simulink model "APPL_DriverFaultDetection"  (R2018b)
settings: configuration reference "CodeConfig_10_ms" (kept outside this file)
undefined symbols (not defined in the file): CAL_LockErrNoTime_30ms, CAL_ManualSwValid_90s, CAL_MotorHallInvalid_2s, CAL_MotorMaxRunTime_60s, CAL_MotorRelayErr_2s, CAL_MotorStall_750ms, D_DrSoftStopDef_B, D_DrSoftStopDef_F, D_DrSoftStopDef_H, D_DrSoftStopDef_L, D_Relay_DownBackFault, D_Relay_UpFrontFault, enSeatMoveCmd, FALSE, TRUE
libraries: DareLib x95, simulink x2
(part 2 of 3)

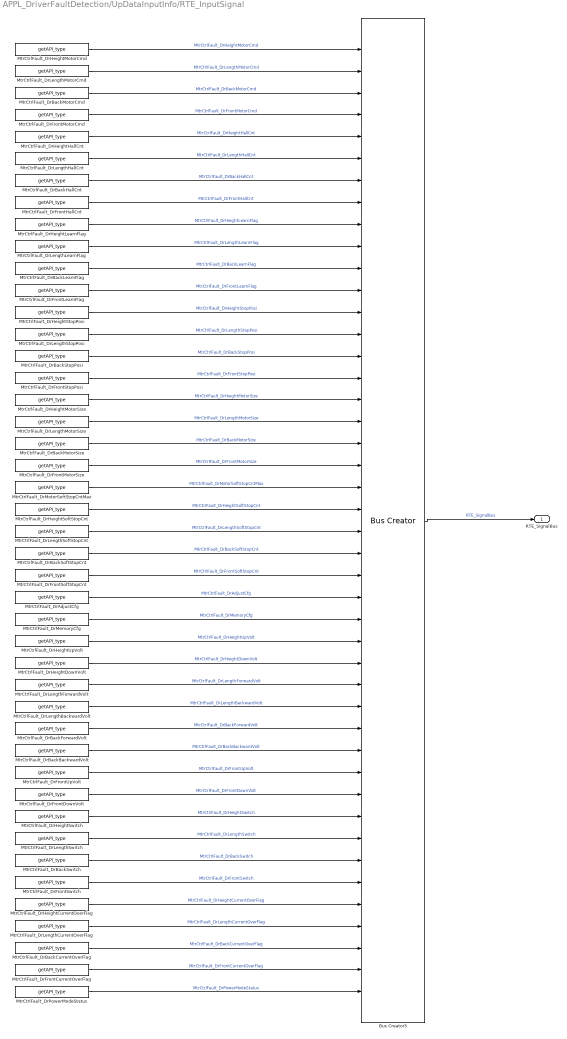
== system APPL_DriverFaultDetection/UpDataInputInfo/RTE_InputSignal ==
  Bus Creator5 : BusCreator  Inputs=44
  MtrCtrlFault_DrAdjustCfg : DareLib/Dare/getAPI_type  g_funcname=Srvl_GetMemIndexDataU8  g_param=EN_MemIndex_DrAdjustConfig  g_type=uint8  g_enum=enDrAdjustEnable  g_size=-1
      settings: AttributesFormatString=%<g_funcname>  SourceProductName=Dare Library
  MtrCtrlFault_DrBackBackwardVolt : DareLib/Dare/getAPI_type  g_funcname=Ecual_GetDrRelayFlagBackBackward  g_param=""  g_type=uint8  g_size=-1
      settings: AttributesFormatString=%<g_funcname>  SourceProductName=Dare Library
  MtrCtrlFault_DrBackCurrentOverFlag : DareLib/Dare/getAPI_type  g_funcname=Ecual_GetDrBackOverCurrentFlag  g_param=""  g_type=uint8  g_size=-1
      settings: AttributesFormatString=%<g_funcname>  SourceProductName=Dare Library
  MtrCtrlFault_DrBackForwardVolt : DareLib/Dare/getAPI_type  g_funcname=Ecual_GetDrRelayFlagBackForward  g_param=""  g_type=uint8  g_size=-1
      settings: AttributesFormatString=%<g_funcname>  SourceProductName=Dare Library
  MtrCtrlFault_DrBackHallCnt : DareLib/Dare/getAPI_type  g_funcname=Cdd_GetCurrentHallCnt  g_param=EN_DriverBack  g_type=uint16  g_size=-1
      settings: AttributesFormatString=%<g_funcname>  SourceProductName=Dare Library
  MtrCtrlFault_DrBackLearnFlag : DareLib/Dare/getAPI_type  g_funcname=Cdd_GetMotorLearnFlag  g_param=EN_DriverBack  g_type=uint8  g_size=-1
      settings: AttributesFormatString=%<g_funcname>  SourceProductName=Dare Library
  MtrCtrlFault_DrBackMotorCmd : DareLib/Dare/getAPI_type  g_funcname=Rte_GetVfb_DrBackMotorCmd  g_param=""  g_type=uint8  g_size=-1
      settings: AttributesFormatString=%<g_funcname>  SourceProductName=Dare Library
  MtrCtrlFault_DrBackMotorSize : DareLib/Dare/getAPI_type  g_funcname=Cdd_GetMotorSize  g_param=EN_DriverBack  g_type=uint16  g_size=-1
      settings: AttributesFormatString=%<g_funcname>  SourceProductName=Dare Library
  MtrCtrlFault_DrBackSoftStopCnt : DareLib/Dare/getAPI_type  g_funcname=Srvl_GetMemIndexDataU8  g_param=EN_MemIndex_DrBackSoftStopCnt  g_type=uint8  g_size=-1
      settings: AttributesFormatString=%<g_funcname>  SourceProductName=Dare Library
  MtrCtrlFault_DrBackStopPosi : DareLib/Dare/getAPI_type  g_funcname=Cdd_GetMotorHardStop  g_param=EN_DriverBack  g_type=uint16  g_size=-1
      settings: AttributesFormatString=%<g_funcname>  SourceProductName=Dare Library
  MtrCtrlFault_DrBackSwitch : DareLib/Dare/getAPI_type  g_funcname=Ecual_GetDrBackSwitchCmd  g_param=""  g_type=uint8  g_enum=enSeatMoveCmd  g_size=-1
      settings: AttributesFormatString=%<g_funcname>  SourceProductName=Dare Library
  MtrCtrlFault_DrFrontCurrentOverFlag : DareLib/Dare/getAPI_type  g_funcname=Ecual_GetDrFrontOverCurrentFlag  g_param=""  g_type=uint8  g_size=-1
      settings: AttributesFormatString=%<g_funcname>  SourceProductName=Dare Library
  MtrCtrlFault_DrFrontDownVolt : DareLib/Dare/getAPI_type  g_funcname=Ecual_GetDrRelayFlagFrontDown  g_param=""  g_type=uint8  g_size=-1
      settings: AttributesFormatString=%<g_funcname>  SourceProductName=Dare Library
  MtrCtrlFault_DrFrontHallCnt : DareLib/Dare/getAPI_type  g_funcname=Cdd_GetCurrentHallCnt  g_param=EN_DriverFront  g_type=uint16  g_size=-1
      settings: AttributesFormatString=%<g_funcname>  SourceProductName=Dare Library
  MtrCtrlFault_DrFrontLearnFlag : DareLib/Dare/getAPI_type  g_funcname=Cdd_GetMotorLearnFlag  g_param=EN_DriverFront  g_type=uint8  g_size=-1
      settings: AttributesFormatString=%<g_funcname>  SourceProductName=Dare Library
  MtrCtrlFault_DrFrontMotorCmd : DareLib/Dare/getAPI_type  g_funcname=Rte_GetVfb_DrFrontMotorCmd  g_param=""  g_type=uint8  g_size=-1
      settings: AttributesFormatString=%<g_funcname>  SourceProductName=Dare Library
  MtrCtrlFault_DrFrontMotorSize : DareLib/Dare/getAPI_type  g_funcname=Cdd_GetMotorSize  g_param=EN_DriverFront  g_type=uint16  g_size=-1
      settings: AttributesFormatString=%<g_funcname>  SourceProductName=Dare Library
  MtrCtrlFault_DrFrontSoftStopCnt : DareLib/Dare/getAPI_type  g_funcname=Srvl_GetMemIndexDataU8  g_param=EN_MemIndex_DrFrontSoftStopCnt  g_type=uint8  g_size=-1
      settings: AttributesFormatString=%<g_funcname>  SourceProductName=Dare Library
  MtrCtrlFault_DrFrontStopPosi : DareLib/Dare/getAPI_type  g_funcname=Cdd_GetMotorHardStop  g_param=EN_DriverFront  g_type=uint16  g_size=-1
      settings: AttributesFormatString=%<g_funcname>  SourceProductName=Dare Library
  MtrCtrlFault_DrFrontSwitch : DareLib/Dare/getAPI_type  g_funcname=Ecual_GetDrFrontSwitchCmd  g_param=""  g_type=uint8  g_enum=enSeatMoveCmd  g_size=-1
      settings: AttributesFormatString=%<g_funcname>  SourceProductName=Dare Library
  MtrCtrlFault_DrFrontUpVolt : DareLib/Dare/getAPI_type  g_funcname=Ecual_GetDrRelayFlagFrontUp  g_param=""  g_type=uint8  g_size=-1
      settings: AttributesFormatString=%<g_funcname>  SourceProductName=Dare Library
  MtrCtrlFault_DrHeightCurrentOverFlag : DareLib/Dare/getAPI_type  g_funcname=Ecual_GetDrHeightOverCurrentFlag  g_param=""  g_type=uint8  g_size=-1
      settings: AttributesFormatString=%<g_funcname>  SourceProductName=Dare Library
  MtrCtrlFault_DrHeightDownVolt : DareLib/Dare/getAPI_type  g_funcname=Ecual_GetDrRelayFlagHeightDN  g_param=""  g_type=uint8  g_size=-1
      settings: AttributesFormatString=%<g_funcname>  SourceProductName=Dare Library
  MtrCtrlFault_DrHeightHallCnt : DareLib/Dare/getAPI_type  g_funcname=Cdd_GetCurrentHallCnt  g_param=EN_DriverHeight  g_type=uint16  g_size=-1
      settings: AttributesFormatString=%<g_funcname>  SourceProductName=Dare Library
  MtrCtrlFault_DrHeightLearnFlag : DareLib/Dare/getAPI_type  g_funcname=Cdd_GetMotorLearnFlag  g_param=EN_DriverHeight  g_type=uint8  g_size=-1
      settings: AttributesFormatString=%<g_funcname>  SourceProductName=Dare Library
  MtrCtrlFault_DrHeightMotorCmd : DareLib/Dare/getAPI_type  g_funcname=Rte_GetVfb_DrHeightMotorCmd  g_param=""  g_type=uint8  g_size=-1
      settings: AttributesFormatString=%<g_funcname>  SourceProductName=Dare Library
  MtrCtrlFault_DrHeightMotorSize : DareLib/Dare/getAPI_type  g_funcname=Cdd_GetMotorSize  g_param=EN_DriverHeight  g_type=uint16  g_size=-1
      settings: AttributesFormatString=%<g_funcname>  SourceProductName=Dare Library
  MtrCtrlFault_DrHeightSoftStopCnt : DareLib/Dare/getAPI_type  g_funcname=Srvl_GetMemIndexDataU8  g_param=EN_MemIndex_DrHeightSoftStopCnt  g_type=uint8  g_size=-1
      settings: AttributesFormatString=%<g_funcname>  SourceProductName=Dare Library
  MtrCtrlFault_DrHeightStopPosi : DareLib/Dare/getAPI_type  g_funcname=Cdd_GetMotorHardStop  g_param=EN_DriverHeight  g_type=uint16  g_size=-1
      settings: AttributesFormatString=%<g_funcname>  SourceProductName=Dare Library
  MtrCtrlFault_DrHeightSwitch : DareLib/Dare/getAPI_type  g_funcname=Ecual_GetDrHeightSwitchCmd  g_param=""  g_type=uint8  g_enum=enSeatMoveCmd  g_size=-1
      settings: AttributesFormatString=%<g_funcname>  SourceProductName=Dare Library
  MtrCtrlFault_DrHeightUpVolt : DareLib/Dare/getAPI_type  g_funcname=Ecual_GetDrRelayFlagHeightUp  g_param=""  g_type=uint8  g_size=-1
      settings: AttributesFormatString=%<g_funcname>  SourceProductName=Dare Library
  MtrCtrlFault_DrLengthBackwardVolt : DareLib/Dare/getAPI_type  g_funcname=Ecual_GetDrRelayFlagLenghtBackward  g_param=""  g_type=uint8  g_size=-1
      settings: AttributesFormatString=%<g_funcname>  SourceProductName=Dare Library
  MtrCtrlFault_DrLengthCurrentOverFlag : DareLib/Dare/getAPI_type  g_funcname=Ecual_GetDrLengthOverCurrentFlag  g_param=""  g_type=uint8  g_size=-1
      settings: AttributesFormatString=%<g_funcname>  SourceProductName=Dare Library
  MtrCtrlFault_DrLengthForwardVolt : DareLib/Dare/getAPI_type  g_funcname=Ecual_GetDrRelayFlagLenghtForward  g_param=""  g_type=uint8  g_size=-1
      settings: AttributesFormatString=%<g_funcname>  SourceProductName=Dare Library
  MtrCtrlFault_DrLengthHallCnt : DareLib/Dare/getAPI_type  g_funcname=Cdd_GetCurrentHallCnt  g_param=EN_DriverLength  g_type=uint16  g_size=-1
      settings: AttributesFormatString=%<g_funcname>  SourceProductName=Dare Library
  MtrCtrlFault_DrLengthLearnFlag : DareLib/Dare/getAPI_type  g_funcname=Cdd_GetMotorLearnFlag  g_param=EN_DriverLength  g_type=uint8  g_size=-1
      settings: AttributesFormatString=%<g_funcname>  SourceProductName=Dare Library
  MtrCtrlFault_DrLengthMotorCmd : DareLib/Dare/getAPI_type  g_funcname=Rte_GetVfb_DrLengthMotorCmd  g_param=""  g_type=uint8  g_size=-1
      settings: AttributesFormatString=%<g_funcname>  SourceProductName=Dare Library
  MtrCtrlFault_DrLengthMotorSize : DareLib/Dare/getAPI_type  g_funcname=Cdd_GetMotorSize  g_param=EN_DriverLength  g_type=uint16  g_size=-1
      settings: AttributesFormatString=%<g_funcname>  SourceProductName=Dare Library
  MtrCtrlFault_DrLengthSoftStopCnt : DareLib/Dare/getAPI_type  g_funcname=Srvl_GetMemIndexDataU8  g_param=EN_MemIndex_DrLengthSoftStopCnt  g_type=uint8  g_size=-1
      settings: AttributesFormatString=%<g_funcname>  SourceProductName=Dare Library
  MtrCtrlFault_DrLengthStopPosi : DareLib/Dare/getAPI_type  g_funcname=Cdd_GetMotorHardStop  g_param=EN_DriverLength  g_type=uint16  g_size=-1
      settings: AttributesFormatString=%<g_funcname>  SourceProductName=Dare Library
  MtrCtrlFault_DrLengthSwitch : DareLib/Dare/getAPI_type  g_funcname=Ecual_GetDrLengthSwitchCmd  g_param=""  g_type=uint8  g_enum=enSeatMoveCmd  g_size=-1
      settings: AttributesFormatString=%<g_funcname>  SourceProductName=Dare Library
  MtrCtrlFault_DrMemoryCfg : DareLib/Dare/getAPI_type  g_funcname=Srvl_GetMemIndexDataU8  g_param=EN_MemIndex_DrMemoryConfig  g_type=uint8  g_size=-1
      settings: AttributesFormatString=%<g_funcname>  SourceProductName=Dare Library
  MtrCtrlFault_DrMotorSoftStopCntMax : DareLib/Dare/getAPI_type  g_funcname=Srvl_GetMemIndexDataU8  g_param=EN_MemIndex_MotorSoftStopCntMax  g_type=uint8  g_size=-1
      settings: AttributesFormatString=%<g_funcname>  SourceProductName=Dare Library
  MtrCtrlFault_DrPowerModeStatus : DareLib/Dare/getAPI_type  g_funcname=Rte_GetVfb_PowerMode  g_param=""  g_type=uint8  g_enum=enIgnSts  g_size=-1
      settings: AttributesFormatString=%<g_funcname>  SourceProductName=Dare Library
  RTE_SignalBus : Outport
  wires:
  Bus Creator5/1 -> RTE_SignalBus/1  "RTE_SignalBus"
  MtrCtrlFault_DrHeightMotorCmd/1 -> Bus Creator5/1  "MtrCtrlFault_DrHeightMotorCmd"
  MtrCtrlFault_DrLengthMotorCmd/1 -> Bus Creator5/2  "MtrCtrlFault_DrLengthMotorCmd"
  MtrCtrlFault_DrBackMotorCmd/1 -> Bus Creator5/3  "MtrCtrlFault_DrBackMotorCmd"
  MtrCtrlFault_DrFrontMotorCmd/1 -> Bus Creator5/4  "MtrCtrlFault_DrFrontMotorCmd"
  MtrCtrlFault_DrHeightHallCnt/1 -> Bus Creator5/5  "MtrCtrlFault_DrHeightHallCnt"
  MtrCtrlFault_DrLengthHallCnt/1 -> Bus Creator5/6  "MtrCtrlFault_DrLengthHallCnt"
  MtrCtrlFault_DrBackHallCnt/1 -> Bus Creator5/7  "MtrCtrlFault_DrBackHallCnt"
  MtrCtrlFault_DrFrontHallCnt/1 -> Bus Creator5/8  "MtrCtrlFault_DrFrontHallCnt"
  MtrCtrlFault_DrHeightLearnFlag/1 -> Bus Creator5/9  "MtrCtrlFault_DrHeightLearnFlag"
  MtrCtrlFault_DrLengthLearnFlag/1 -> Bus Creator5/10  "MtrCtrlFault_DrLengthLearnFlag"
  MtrCtrlFault_DrBackLearnFlag/1 -> Bus Creator5/11  "MtrCtrlFault_DrBackLearnFlag"
  MtrCtrlFault_DrFrontLearnFlag/1 -> Bus Creator5/12  "MtrCtrlFault_DrFrontLearnFlag"
  MtrCtrlFault_DrHeightStopPosi/1 -> Bus Creator5/13  "MtrCtrlFault_DrHeightStopPosi"
  MtrCtrlFault_DrLengthStopPosi/1 -> Bus Creator5/14  "MtrCtrlFault_DrLengthStopPosi"
  MtrCtrlFault_DrBackStopPosi/1 -> Bus Creator5/15  "MtrCtrlFault_DrBackStopPosi"
  MtrCtrlFault_DrFrontStopPosi/1 -> Bus Creator5/16  "MtrCtrlFault_DrFrontStopPosi"
  MtrCtrlFault_DrHeightMotorSize/1 -> Bus Creator5/17  "MtrCtrlFault_DrHeightMotorSize"
  MtrCtrlFault_DrLengthMotorSize/1 -> Bus Creator5/18  "MtrCtrlFault_DrLengthMotorSize"
  MtrCtrlFault_DrBackMotorSize/1 -> Bus Creator5/19  "MtrCtrlFault_DrBackMotorSize"
  MtrCtrlFault_DrFrontMotorSize/1 -> Bus Creator5/20  "MtrCtrlFault_DrFrontMotorSize"
  MtrCtrlFault_DrMotorSoftStopCntMax/1 -> Bus Creator5/21  "MtrCtrlFault_DrMotorSoftStopCntMax"
  MtrCtrlFault_DrHeightSoftStopCnt/1 -> Bus Creator5/22  "MtrCtrlFault_DrHeightSoftStopCnt"
  MtrCtrlFault_DrLengthSoftStopCnt/1 -> Bus Creator5/23  "MtrCtrlFault_DrLengthSoftStopCnt"
  MtrCtrlFault_DrBackSoftStopCnt/1 -> Bus Creator5/24  "MtrCtrlFault_DrBackSoftStopCnt"
  MtrCtrlFault_DrFrontSoftStopCnt/1 -> Bus Creator5/25  "MtrCtrlFault_DrFrontSoftStopCnt"
  MtrCtrlFault_DrAdjustCfg/1 -> Bus Creator5/26  "MtrCtrlFault_DrAdjustCfg"
  MtrCtrlFault_DrMemoryCfg/1 -> Bus Creator5/27  "MtrCtrlFault_DrMemoryCfg"
  MtrCtrlFault_DrHeightUpVolt/1 -> Bus Creator5/28  "MtrCtrlFault_DrHeightUpVolt"
  MtrCtrlFault_DrHeightDownVolt/1 -> Bus Creator5/29  "MtrCtrlFault_DrHeightDownVolt"
  MtrCtrlFault_DrLengthForwardVolt/1 -> Bus Creator5/30  "MtrCtrlFault_DrLengthForwardVolt"
  MtrCtrlFault_DrLengthBackwardVolt/1 -> Bus Creator5/31  "MtrCtrlFault_DrLengthBackwardVolt"
  MtrCtrlFault_DrBackForwardVolt/1 -> Bus Creator5/32  "MtrCtrlFault_DrBackForwardVolt"
  MtrCtrlFault_DrBackBackwardVolt/1 -> Bus Creator5/33  "MtrCtrlFault_DrBackBackwardVolt"
  MtrCtrlFault_DrFrontUpVolt/1 -> Bus Creator5/34  "MtrCtrlFault_DrFrontUpVolt"
  MtrCtrlFault_DrFrontDownVolt/1 -> Bus Creator5/35  "MtrCtrlFault_DrFrontDownVolt"
  MtrCtrlFault_DrHeightSwitch/1 -> Bus Creator5/36  "MtrCtrlFault_DrHeightSwitch"
  MtrCtrlFault_DrLengthSwitch/1 -> Bus Creator5/37  "MtrCtrlFault_DrLengthSwitch"
  MtrCtrlFault_DrBackSwitch/1 -> Bus Creator5/38  "MtrCtrlFault_DrBackSwitch"
  MtrCtrlFault_DrFrontSwitch/1 -> Bus Creator5/39  "MtrCtrlFault_DrFrontSwitch"
  MtrCtrlFault_DrHeightCurrentOverFlag/1 -> Bus Creator5/40  "MtrCtrlFault_DrHeightCurrentOverFlag"
  MtrCtrlFault_DrLengthCurrentOverFlag/1 -> Bus Creator5/41  "MtrCtrlFault_DrLengthCurrentOverFlag"
  MtrCtrlFault_DrBackCurrentOverFlag/1 -> Bus Creator5/42  "MtrCtrlFault_DrBackCurrentOverFlag"
  MtrCtrlFault_DrFrontCurrentOverFlag/1 -> Bus Creator5/43  "MtrCtrlFault_DrFrontCurrentOverFlag"
  MtrCtrlFault_DrPowerModeStatus/1 -> Bus Creator5/44  "MtrCtrlFault_DrPowerModeStatus"

== system APPL_DriverFaultDetection/LogicCtrl/AdheAndEffec/SwitchErrorDetection/GetCurMsTs ==
  f : TriggerPort  TriggerType=function-call  VariantControl=(inherit)
      settings: CopyFcn=Stateflow.SLINSF.SimulinkMan.removeBlockPreDeleteFcn  PreDeleteFcn=Stateflow.SLINSF.SimulinkMan.unsafePredeleteFcn
  DrAdj_LenAdjSize : DareLib/Dare/getAPI_type  g_funcname=D_HAL_GET_CUR_MS_TS  g_param=""  g_type=uint32  g_size=-1
      settings: SourceProductName=Dare Library
  Ts : Outport
  wires:
  DrAdj_LenAdjSize/1 -> Ts/1  "DrAdj_CurMsTs"

== system APPL_DriverFaultDetection/LogicCtrl/AdheAndEffec/SwitchErrorDetection/GetDefTime ==
  DefTs : Inport
  Ts : Inport  Port=2
  f : TriggerPort  TriggerType=function-call  VariantControl=(inherit)
      settings: CopyFcn=Stateflow.SLINSF.SimulinkMan.removeBlockPreDeleteFcn  PreDeleteFcn=Stateflow.SLINSF.SimulinkMan.unsafePredeleteFcn
  Chart : Stateflow chart  TreatAsAtomicUnit=on
  OutTs : Outport
  wires:
  DefTs/1 -> Chart/1(DefTs)
  Ts/1 -> Chart/2(Ts)
  Chart/1(OutTs) -> OutTs/1

== system APPL_DriverFaultDetection/LogicCtrl/AdheAndEffec/SwitchErrorDetection/TimeDiffTs ==
  lastTs : Inport
  Ts : Inport  Port=2
  f : TriggerPort  TriggerType=function-call  VariantControl=(inherit)
      settings: CopyFcn=Stateflow.SLINSF.SimulinkMan.removeBlockPreDeleteFcn  PreDeleteFcn=Stateflow.SLINSF.SimulinkMan.unsafePredeleteFcn
  Chart : Stateflow chart  TreatAsAtomicUnit=on
  OutTs : Outport
  wires:
  lastTs/1 -> Chart/1(lastTs)
  Ts/1 -> Chart/2(Ts)
  Chart/1(OutTs) -> OutTs/1

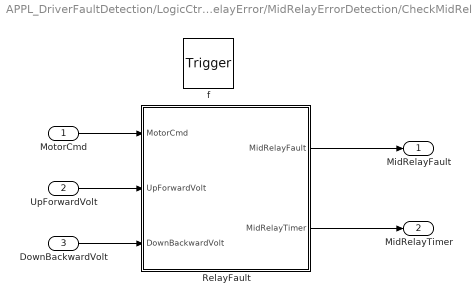
== system APPL_DriverFaultDetection/LogicCtrl/RelayError/MidRelayErrorDetection/CheckMidRelayFault ==
  MotorCmd : Inport  OutDataTypeStr=uint8  PortDimensions=1
  UpForwardVolt : Inport  Port=2  OutDataTypeStr=uint8  PortDimensions=1
  DownBackwardVolt : Inport  Port=3  OutDataTypeStr=uint8  PortDimensions=1
  f : TriggerPort  TriggerType=function-call  VariantControl=(inherit)
      settings: CopyFcn=Stateflow.SLINSF.SimulinkMan.removeBlockPreDeleteFcn  PreDeleteFcn=Stateflow.SLINSF.SimulinkMan.unsafePredeleteFcn
  RelayFault : Stateflow chart  TreatAsAtomicUnit=on
  MidRelayFault : Outport  OutDataTypeStr=uint8
  MidRelayTimer : Outport  Port=2  OutDataTypeStr=uint8
  wires:
  MotorCmd/1 -> RelayFault/1(MotorCmd)
  UpForwardVolt/1 -> RelayFault/2(UpForwardVolt)
  DownBackwardVolt/1 -> RelayFault/3(DownBackwardVolt)
  RelayFault/1(MidRelayFault) -> MidRelayFault/1
  RelayFault/2(MidRelayTimer) -> MidRelayTimer/1

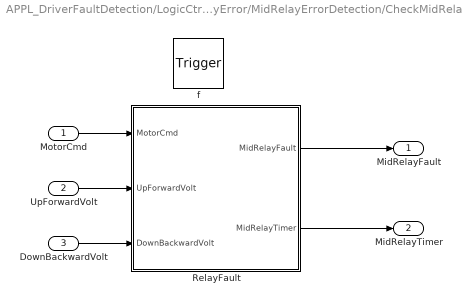
== system APPL_DriverFaultDetection/LogicCtrl/RelayError/MidRelayErrorDetection/CheckMidRelayFault1 ==
  MotorCmd : Inport  OutDataTypeStr=uint8  PortDimensions=1
  UpForwardVolt : Inport  Port=2  OutDataTypeStr=uint8  PortDimensions=1
  DownBackwardVolt : Inport  Port=3  OutDataTypeStr=uint8  PortDimensions=1
  f : TriggerPort  TriggerType=function-call  VariantControl=(inherit)
      settings: CopyFcn=Stateflow.SLINSF.SimulinkMan.removeBlockPreDeleteFcn  PreDeleteFcn=Stateflow.SLINSF.SimulinkMan.unsafePredeleteFcn
  RelayFault : Stateflow chart  TreatAsAtomicUnit=on
  MidRelayFault : Outport  OutDataTypeStr=uint8
  MidRelayTimer : Outport  Port=2  OutDataTypeStr=uint8
  wires:
  MotorCmd/1 -> RelayFault/1(MotorCmd)
  UpForwardVolt/1 -> RelayFault/2(UpForwardVolt)
  DownBackwardVolt/1 -> RelayFault/3(DownBackwardVolt)
  RelayFault/1(MidRelayFault) -> MidRelayFault/1
  RelayFault/2(MidRelayTimer) -> MidRelayTimer/1

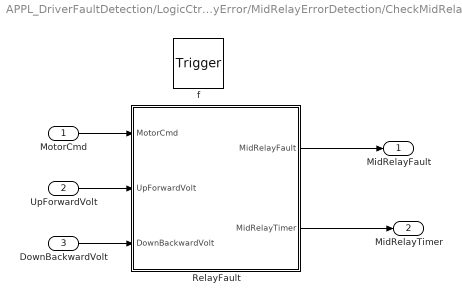
== system APPL_DriverFaultDetection/LogicCtrl/RelayError/MidRelayErrorDetection/CheckMidRelayFault2 ==
  MotorCmd : Inport  OutDataTypeStr=uint8  PortDimensions=1
  UpForwardVolt : Inport  Port=2  OutDataTypeStr=uint8  PortDimensions=1
  DownBackwardVolt : Inport  Port=3  OutDataTypeStr=uint8  PortDimensions=1
  f : TriggerPort  TriggerType=function-call  VariantControl=(inherit)
      settings: CopyFcn=Stateflow.SLINSF.SimulinkMan.removeBlockPreDeleteFcn  PreDeleteFcn=Stateflow.SLINSF.SimulinkMan.unsafePredeleteFcn
  RelayFault : Stateflow chart  TreatAsAtomicUnit=on
  MidRelayFault : Outport  OutDataTypeStr=uint8
  MidRelayTimer : Outport  Port=2  OutDataTypeStr=uint8
  wires:
  MotorCmd/1 -> RelayFault/1(MotorCmd)
  UpForwardVolt/1 -> RelayFault/2(UpForwardVolt)
  DownBackwardVolt/1 -> RelayFault/3(DownBackwardVolt)
  RelayFault/1(MidRelayFault) -> MidRelayFault/1
  RelayFault/2(MidRelayTimer) -> MidRelayTimer/1

== system APPL_DriverFaultDetection/LogicCtrl/RelayError/MidRelayErrorDetection/CheckMidRelayFault3 ==
  MotorCmd : Inport  OutDataTypeStr=uint8  PortDimensions=1
  UpForwardVolt : Inport  Port=2  OutDataTypeStr=uint8  PortDimensions=1
  DownBackwardVolt : Inport  Port=3  OutDataTypeStr=uint8  PortDimensions=1
  f : TriggerPort  TriggerType=function-call  VariantControl=(inherit)
      settings: CopyFcn=Stateflow.SLINSF.SimulinkMan.removeBlockPreDeleteFcn  PreDeleteFcn=Stateflow.SLINSF.SimulinkMan.unsafePredeleteFcn
  RelayFault : Stateflow chart  TreatAsAtomicUnit=on
  MidRelayFault : Outport  OutDataTypeStr=uint8
  MidRelayTimer : Outport  Port=2  OutDataTypeStr=uint8
  wires:
  MotorCmd/1 -> RelayFault/1(MotorCmd)
  UpForwardVolt/1 -> RelayFault/2(UpForwardVolt)
  DownBackwardVolt/1 -> RelayFault/3(DownBackwardVolt)
  RelayFault/1(MidRelayFault) -> MidRelayFault/1
  RelayFault/2(MidRelayTimer) -> MidRelayTimer/1

== system APPL_DriverFaultDetection/LogicCtrl/SoftStopPoint/SoftStopPointDetection/DrAdj_SetBackSoftStopCnt ==
  Cnt : Inport
  f : TriggerPort  TriggerType=function-call  VariantControl=(inherit)
      settings: CopyFcn=Stateflow.SLINSF.SimulinkMan.removeBlockPreDeleteFcn  PreDeleteFcn=Stateflow.SLINSF.SimulinkMan.unsafePredeleteFcn
  DriverFrontMoveType12 : DareLib/Dare/setAPI_type  g_funcname=Srvl_SetMemIndexDataU8  g_param=EN_MemIndex_DrBackSoftStopCnt  g_type=uint8  g_size=-1
      settings: AttributesFormatString=%<g_funcname>  SourceProductName=Dare Library
  wires:
  Cnt/1 -> DriverFrontMoveType12/1

== system APPL_DriverFaultDetection/LogicCtrl/SoftStopPoint/SoftStopPointDetection/DrAdj_SetFrontSoftStopCnt ==
  Cnt : Inport
  f : TriggerPort  TriggerType=function-call  VariantControl=(inherit)
      settings: CopyFcn=Stateflow.SLINSF.SimulinkMan.removeBlockPreDeleteFcn  PreDeleteFcn=Stateflow.SLINSF.SimulinkMan.unsafePredeleteFcn
  DriverFrontMoveType12 : DareLib/Dare/setAPI_type  g_funcname=Srvl_SetMemIndexDataU8  g_param=EN_MemIndex_DrFrontSoftStopCnt  g_type=uint8  g_size=-1
      settings: AttributesFormatString=%<g_funcname>  SourceProductName=Dare Library
  wires:
  Cnt/1 -> DriverFrontMoveType12/1

== system APPL_DriverFaultDetection/LogicCtrl/SoftStopPoint/SoftStopPointDetection/DrAdj_SetHeightSoftStopCnt ==
  Cnt : Inport
  f : TriggerPort  TriggerType=function-call  VariantControl=(inherit)
      settings: CopyFcn=Stateflow.SLINSF.SimulinkMan.removeBlockPreDeleteFcn  PreDeleteFcn=Stateflow.SLINSF.SimulinkMan.unsafePredeleteFcn
  DriverFrontMoveType12 : DareLib/Dare/setAPI_type  g_funcname=Srvl_SetMemIndexDataU8  g_param=EN_MemIndex_DrHeightSoftStopCnt  g_type=uint8  g_size=-1
      settings: AttributesFormatString=%<g_funcname>  SourceProductName=Dare Library
  wires:
  Cnt/1 -> DriverFrontMoveType12/1

== system APPL_DriverFaultDetection/LogicCtrl/SoftStopPoint/SoftStopPointDetection/DrAdj_SetLengthSoftStopCnt ==
  Cnt : Inport
  f : TriggerPort  TriggerType=function-call  VariantControl=(inherit)
      settings: CopyFcn=Stateflow.SLINSF.SimulinkMan.removeBlockPreDeleteFcn  PreDeleteFcn=Stateflow.SLINSF.SimulinkMan.unsafePredeleteFcn
  DriverFrontMoveType12 : DareLib/Dare/setAPI_type  g_funcname=Srvl_SetMemIndexDataU8  g_param=EN_MemIndex_DrLengthSoftStopCnt  g_type=uint8  g_size=-1
      settings: AttributesFormatString=%<g_funcname>  SourceProductName=Dare Library
  wires:
  Cnt/1 -> DriverFrontMoveType12/1

== stateflow chart APPL_DriverFaultDetection/LogicCtrl/SwitchErrDeal/ SWProcess  ==
  settings: description=硬线开关信号处理 SWProcess
  state DSM_SWAdjust
    state HeightSWProcess [parallel]
      settings: executionOrder=1
      state Enable
        en:
        CurrentHeightSwCmd =DrMtr_HeightSwitchCmd;
        du:
        CurrentHeightSwCmd =DrMtr_HeightSwitchCmd;
      state Disable
        en:
        CurrentHeightSwCmd = FALSE;
      (default) -> DSM_SWAdjust.HeightSWProcess.Disable
      DSM_SWAdjust.HeightSWProcess.Disable -> DSM_SWAdjust.HeightSWProcess.Enable : /* 高度本地开关命令故障处理 */
          | [DrMtr_HeightSwitchCmd !=FALSE ...
          | &&FALSE == DrMtr_HeightSwitchAdheErr ...
          | && FALSE ==DrMtr_HeightRelayAdhesionErr ...
          | &&FALSE == DrMtr_HeightStallErr]
      DSM_SWAdjust.HeightSWProcess.Enable -> DSM_SWAdjust.HeightSWProcess.Disable : [DrMtr_HeightSwitchCmd ==FALSE ...
          | || FALSE != DrMtr_HeightSwitchAdheErr ...
          | || TRUE == DrMtr_HeightRelayAdhesionErr ...
          | || TRUE == DrMtr_HeightStallErr]
    state LengthSWProcess [parallel]
      settings: executionOrder=2
      state Enable
        en:
        CurrentLengthSwCmd =DrMtr_LengthSwitchCmd;
        du:
        CurrentLengthSwCmd =DrMtr_LengthSwitchCmd;
      state Disable
        en:
        CurrentLengthSwCmd = FALSE;
      (default) -> DSM_SWAdjust.LengthSWProcess.Disable
      DSM_SWAdjust.LengthSWProcess.Disable -> DSM_SWAdjust.LengthSWProcess.Enable : /* 纵向本地开关命令故障处理 */
          | [DrMtr_LengthSwitchCmd !=FALSE ...
          | &&FALSE == DrMtr_LengthSwitchAdheErr...
          | && FALSE ==DrMtr_LengthRelayAdhesionErr ...
          | &&FALSE == DrMtr_LengthStallErr]
      DSM_SWAdjust.LengthSWProcess.Enable -> DSM_SWAdjust.LengthSWProcess.Disable : [DrMtr_LengthSwitchCmd ==FALSE ...
          | || FALSE !=  DrMtr_LengthSwitchAdheErr...
          | || TRUE == DrMtr_LengthRelayAdhesionErr ...
          | || TRUE == DrMtr_LengthStallErr]
    state BackSWProcess [parallel]
      settings: executionOrder=3
      state Enable
        en:
        CurrentBackSwCmd =DrMtr_BackSwitchCmd;
        du:
        CurrentBackSwCmd =DrMtr_BackSwitchCmd;
      state Disable
        en:
        CurrentBackSwCmd = FALSE;
      (default) -> DSM_SWAdjust.BackSWProcess.Disable
      DSM_SWAdjust.BackSWProcess.Disable -> DSM_SWAdjust.BackSWProcess.Enable : /* 靠背本地开关命令故障处理 */
          | [DrMtr_BackSwitchCmd !=FALSE ...
          | &&FALSE == DrMtr_BackRelayAdhesionErr ...
          | &&FALSE == DrMtr_BackSwitchAdheErr...
          | &&FALSE == DrMtr_BackStallErr]
      DSM_SWAdjust.BackSWProcess.Enable -> DSM_SWAdjust.BackSWProcess.Disable : [DrMtr_BackSwitchCmd ==FALSE ...
          | || FALSE != DrMtr_BackRelayAdhesionErr ...
          | || TRUE == DrMtr_BackSwitchAdheErr...
          | || TRUE == DrMtr_BackStallErr]
    state FrontSWProcess [parallel]
      settings: executionOrder=4
      state Enable
        en:
        CurrentFrontSwCmd =DrMtr_FrontSwitchCmd;
        du:
        CurrentFrontSwCmd =DrMtr_FrontSwitchCmd;
      state Disable
        en:
        CurrentFrontSwCmd = FALSE;
      (default) -> DSM_SWAdjust.FrontSWProcess.Disable
      DSM_SWAdjust.FrontSWProcess.Disable -> DSM_SWAdjust.FrontSWProcess.Enable : /* 腿托本地开关命令故障处理 && 配置字满足*/
          | [DrMtr_FrontSwitchCmd !=FALSE ...
          | && FALSE == DrMtr_FrontSwitchAdheErr...
          | && FALSE ==DrMtr_FrontRelayAdhesionErr ...
          | && FALSE == DrMtr_FrontStallErr ...
          | && EN_DrTwelveWayMotor == MtrCtrlFault_DrAdjustCfg]
      DSM_SWAdjust.FrontSWProcess.Enable -> DSM_SWAdjust.FrontSWProcess.Disable : [DrMtr_FrontSwitchCmd ==FALSE ...
          | || FALSE !=  DrMtr_FrontSwitchAdheErr...
          | || TRUE == DrMtr_FrontRelayAdhesionErr ...
          | || TRUE == DrMtr_FrontStallErr...
          | || EN_DrTwelveWayMotor != MtrCtrlFault_DrAdjustCfg]
  state Init
    en:
    CurrentHeightSwCmd = FALSE;
    CurrentLengthSwCmd = FALSE;
    CurrentBackSwCmd = FALSE;
    CurrentFrontSwCmd = FALSE;
  (default) -> Init
  Init -> DSM_SWAdjust : /* 非CRANK档位 且非不可调节配置 */
      | [eCrank != MtrCtrlFault_PowerModeStatus ...
      | && (EN_DrSixWayMotor == MtrCtrlFault_DrAdjustCfg ...
      |     || EN_DrTwelveWayMotor == MtrCtrlFault_DrAdjustCfg)]
  DSM_SWAdjust -> Init : /* crank档 或 不可调节配置 */
      | [eCrank == MtrCtrlFault_PowerModeStatus ...
      | || (EN_DrSixWayMotor != MtrCtrlFault_DrAdjustCfg ...
      | && EN_DrTwelveWayMotor != MtrCtrlFault_DrAdjustCfg)]
  data: CurrentHeightSwCmd output Enum: enSeatMoveCmd; CurrentLengthSwCmd output Enum: enSeatMoveCmd; CurrentBackSwCmd output Enum: enSeatMoveCmd; DrMtr_HeightSwitchCmd input; DrMtr_LengthSwitchCmd input; DrMtr_BackSwitchCmd input; DrMtr_FrontSwitchCmd input; DrMtr_HeightRelayAdhesionErr input; DrMtr_LengthRelayAdhesionErr input; DrMtr_BackRelayAdhesionErr input; DrMtr_FrontRelayAdhesionErr input; DrMtr_HeightSwitchAdheErr input; DrMtr_LengthSwitchAdheErr input; DrMtr_BackSwitchAdheErr input; DrMtr_FrontSwitchAdheErr input; CurrentFrontSwCmd output Enum: enSeatMoveCmd; FALSE parameter; TRUE parameter; DrMtr_HeightStallErr input; DrMtr_LengthStallErr input; DrMtr_BackStallErr input; DrMtr_FrontStallErr input; MtrCtrlFault_DrAdjustCfg input; MtrCtrlFault_DrMemoryCfg input; MtrCtrlFault_PowerModeStatus input

== stateflow chart APPL_DriverFaultDetection/LogicCtrl/AdheAndEffec/SwitchErrorDetection/GetDefTime/Chart ==
  (default) -> (junction 3)
  (junction 3) -> (junction 5)
  (junction 5) -> (junction 7) [order 1] : /* 设置比当前小 */
      | [DefTs < Ts]
  (junction 5) -> (junction 13) [order 2] : {OutTs = Ts - DefTs;}
  (junction 7) -> (junction 11) : {OutTs = 0xFFFFFFFF - DefTs;}
  (junction 11) -> (junction 13)
  (junction 13) -> (junction 17)
  data: DefTs input uint32; Ts input uint32; OutTs output uint32

== stateflow chart APPL_DriverFaultDetection/LogicCtrl/RelayError/MidRelayErrorDetection ==
  state [MidRelayFault,MidRelayTimer]  = CheckMidRelayFault(MotorCmd,UpForwardVolt,DownBackwardVolt) [function]
  state [MidRelayFault,MidRelayTimer] = CheckMidRelayFault1(MotorCmd,UpForwardVolt,DownBackwardVolt) [function]
  state [MidRelayFault,MidRelayTimer]  = CheckMidRelayFault2(MotorCmd,UpForwardVolt,DownBackwardVolt) [function]
  state [MidRelayFault,MidRelayTimer]  = CheckMidRelayFault3(MotorCmd,UpForwardVolt,DownBackwardVolt) [function]
  state MidRelayError [parallel]
    settings: executionOrder=1
    (default) -> (junction 66)
    MidRelayError -> (junction 66)
    (junction 66) -> (junction 68) : {[HeightMidRelayFault, HeightMidRelayTimer] = CheckMidRelayFault(MtrCtrlFault_HeightMotorCmd,MtrCtrlFault_HeightUpVolt,MtrCtrlFault_HeightDownVolt);
        | [LengthMidRelayFault, LengthMidRelayTimer] = CheckMidRelayFault1(MtrCtrlFault_LengthMotorCmd,MtrCtrlFault_LengthForwardVolt,MtrCtrlFault_LengthBackwardVolt);
        | [BackMidRelayFault, BackMidRelayTimer] = CheckMidRelayFault2(MtrCtrlFault_BackMotorCmd,MtrCtrlFault_BackForwardVolt,MtrCtrlFault_BackBackwardVolt);
        | [FrontMidRelayFault, FrontMidRelayTimer] = CheckMidRelayFault3(MtrCtrlFault_FrontMotorCmd,MtrCtrlFault_FrontUpVolt,MtrCtrlFault_FrontDownVolt);}
  note: 继电器粘连故障检测
  data: MotorCmd function_input uint8 size=1; UpForwardVolt function_input uint8 size=1; DownBackwardVolt function_input uint8 size=1; MidRelayFault function_output uint8; MidRelayTimer function_output uint8; MotorCmd function_input uint8 size=1; UpForwardVolt function_input uint8 size=1; DownBackwardVolt function_input uint8 size=1; MidRelayFault function_output uint8; MidRelayTimer function_output uint8; MotorCmd function_input uint8 size=1; UpForwardVolt function_input uint8 size=1; DownBackwardVolt function_input uint8 size=1; MidRelayFault function_output uint8; MidRelayTimer function_output uint8; MotorCmd function_input uint8 size=1; UpForwardVolt function_input uint8 size=1; DownBackwardVolt function_input uint8 size=1; MidRelayFault function_output uint8; MidRelayTimer function_output uint8; MtrCtrlFault_HeightUpVolt input uint8; MtrCtrlFault_HeightDownVolt input uint8; MtrCtrlFault_LengthForwardVolt input uint8; MtrCtrlFault_LengthBackwardVolt input uint8; MtrCtrlFault_BackForwardVolt input uint8; MtrCtrlFault_BackBackwardVolt input uint8; MtrCtrlFault_FrontUpVolt input uint8; MtrCtrlFault_FrontDownVolt input uint8; MtrCtrlFault_HeightMotorCmd input uint8; MtrCtrlFault_LengthMotorCmd input uint8; MtrCtrlFault_BackMotorCmd input uint8; MtrCtrlFault_FrontMotorCmd input uint8; HeightMidRelayFault output uint8; LengthMidRelayFault output uint8; BackMidRelayFault output uint8; FrontMidRelayFault output uint8; LengthMidRelayTimer local double; BackMidRelayTimer local double; FrontMidRelayTimer local double; HeightMidRelayTimer local double

== stateflow chart APPL_DriverFaultDetection/LogicCtrl/RelayError/MidRelayErrorDetection/CheckMidRelayFault/RelayFault ==
  state Judge
    ex:
    MidRelayTimer = 0;
    (default) -> (junction 8)
    Judge -> (junction 8) [order 1]
    (junction 8) -> (junction 10) [order 1] : [CAL_MotorRelayErr_2s <= MidRelayTimer]
    (junction 8) -> (junction 14) [order 2] : {MidRelayTimer ++;}
    (junction 10) -> (junction 12) : {MidRelayTimer = CAL_MotorRelayErr_2s;}
    (junction 12) -> (junction 16) [order 1] : [enSeatMoveCmd.EN_UP_FORWARD != MotorCmd ...
        | && FALSE != UpForwardVolt]
    (junction 12) -> (junction 20) [order 2]
    (junction 16) -> (junction 18) : {MidRelayFault = D_Relay_UpFrontFault;}
    (junction 20) -> (junction 23) [order 1] : [enSeatMoveCmd.EN_DN_BACKWARD != MotorCmd ...
        | && FALSE != DownBackwardVolt]
    (junction 20) -> (junction 27) [order 2]
    (junction 23) -> (junction 25) : {MidRelayFault = D_Relay_DownBackFault;}
    (junction 14) -> (junction 27)
    (junction 25) -> (junction 27)
    (junction 18) -> (junction 25)
    (junction 27) -> (junction 31)
  state Normal
    en:
    MidRelayFault = FALSE;
    MidRelayTimer = 0;
  (default) -> Normal
  Normal -> Judge [order 1] : [/*没有输出命令但输出反馈有电压 满足前置条件*/
      | enSeatMoveCmd.EN_NULL == MotorCmd...
      | && (FALSE != UpForwardVolt...
      | || FALSE != DownBackwardVolt)]
  Normal -> Judge [order 2] : [/*输出命令向前/向上命令却有向后/向下电压 */
      | enSeatMoveCmd.EN_UP_FORWARD == MotorCmd...
      | &&  FALSE != DownBackwardVolt]
  Normal -> Judge [order 3] : [/*输出命令向后/向下命令却有向前/向上电压 */
      | enSeatMoveCmd.EN_DN_BACKWARD  == MotorCmd...
      | &&  FALSE != UpForwardVolt]
  Judge -> Normal [order 1] : [/*继电器粘连消失：
      |  1、没有控制开启命令，同时没有电压输出，认为继电器粘连消失
      |  2、控制开启命令，存在对应的电压输出，认为继电器粘连消失*/
      | (enSeatMoveCmd.EN_NULL == MotorCmd...
      | && FALSE == UpForwardVolt...
      | && FALSE == DownBackwardVolt) ...
      | || (enSeatMoveCmd.EN_UP_FORWARD == MotorCmd...
      | && TRUE == UpForwardVolt ...
      | && FALSE == DownBackwardVolt) ...
      | || (enSeatMoveCmd.EN_DN_BACKWARD == MotorCmd ...
      | && FALSE == UpForwardVolt ...
      | && TRUE == DownBackwardVolt) ]
  data: MotorCmd input; UpForwardVolt input; DownBackwardVolt input; MidRelayFault output uint8; CAL_MotorRelayErr_2s parameter; D_Relay_DownBackFault parameter; D_Relay_UpFrontFault parameter; FALSE parameter; TRUE parameter; MidRelayTimer output uint8

== stateflow chart APPL_DriverFaultDetection/LogicCtrl/AdheAndEffec/SwitchErrorDetection ==
  state Ts = GetCurMsTs [function]
  state OutTs = TimeDiffTs(lastTs,Ts) [function]
  state OutTs = GetDefTime(DefTs,Ts) [function]
  state HeightSwitchErrorDeal [parallel]
    settings: executionOrder=1
    state Valid
      (default) -> (junction 280)
      HeightSwitchErrorDeal.Valid -> (junction 280) [order 1]
      (junction 280) -> (junction 282) [order 1] : /*持续有效时间超过90s，则诊断为开关粘滞故障*/
          | [TimeDiffTs(HeightSwTimer,GetCurMsTs()) >= CAL_ManualSwValid_90s]
      (junction 280) -> (junction 286) [order 2] : {HeightSwCmd = MtrCtrlFault_DRHeightSwitch;
          | HeightSwUpAdhesionFault = FALSE;
          | HeightSwDownAdhesionFault = FALSE;}
      (junction 282) -> (junction 407) : {HeightSwCmd = enSeatMoveCmd.EN_NULL;
          | HeightSwTimer = GetDefTime(CAL_ManualSwValid_90s,GetCurMsTs());
          | HeightSwAdhesionFault = TRUE;}
      (junction 407) -> (junction 408) [order 1] : [enSeatMoveCmd.EN_UP_FORWARD == MtrCtrlFault_DRHeightSwitch]
      (junction 407) -> (junction 290) [order 2] : {HeightSwDownAdhesionFault = TRUE;}
      (junction 408) -> (junction 410) : {HeightSwUpAdhesionFault = TRUE;}
      (junction 290) -> (junction 286)
      (junction 410) -> (junction 290)
      (junction 286) -> (junction 300)
    state Invalid
      en:
      HeightSwTimer = GetCurMsTs();
      HeightSwAdhesionFault = FALSE;
      HeightSwCmd = enSeatMoveCmd.EN_NULL;
      HeightSwUpAdhesionFault = FALSE;
      HeightSwDownAdhesionFault = FALSE;
      du:
      HeightSwTimer = GetCurMsTs();
    (default) -> HeightSwitchErrorDeal.Invalid
    HeightSwitchErrorDeal.Invalid -> HeightSwitchErrorDeal.Valid : /*开关有效 */
        | [enSeatMoveCmd.EN_NULL != MtrCtrlFault_DRHeightSwitch]
    HeightSwitchErrorDeal.Valid -> HeightSwitchErrorDeal.Invalid [order 1] : /* 跳变 无效 */
        | [enSeatMoveCmd.EN_NULL == MtrCtrlFault_DRHeightSwitch ...
        | || hasChanged(MtrCtrlFault_DRHeightSwitch)]
  state LengthSwitchErrorDeal [parallel]
    settings: executionOrder=2
    state Valid
      (default) -> (junction 429)
      (junction 429) -> (junction 430) [order 1] : /*持续有效时间超过90s，则诊断为开关粘滞故障*/
          | [TimeDiffTs(LengthSwTimer,GetCurMsTs()) >= CAL_ManualSwValid_90s]
      LengthSwitchErrorDeal.Valid -> (junction 429) [order 1]
      (junction 430) -> (junction 437) : {LengthSwCmd = enSeatMoveCmd.EN_NULL;
          | LengthSwTimer = GetDefTime(CAL_ManualSwValid_90s,GetCurMsTs());
          | LengthSwAdhesionFault = TRUE;}
      (junction 429) -> (junction 436) [order 2] : {LengthSwCmd = MtrCtrlFault_DRLengthSwitch;
          | LengthSwUpAdhesionFault = FALSE;
          | LengthSwDownAdhesionFault = FALSE;}
      (junction 437) -> (junction 442) [order 1] : [enSeatMoveCmd.EN_UP_FORWARD == MtrCtrlFault_DRLengthSwitch]
      (junction 437) -> (junction 433) [order 2] : {LengthSwDownAdhesionFault = TRUE;}
      (junction 442) -> (junction 441) : {LengthSwUpAdhesionFault = TRUE;}
      (junction 441) -> (junction 433)
      (junction 433) -> (junction 436)
      (junction 436) -> (junction 435)
    state Invalid
      en:
      LengthSwTimer = GetCurMsTs();
      LengthSwAdhesionFault = FALSE;
      LengthSwCmd = enSeatMoveCmd.EN_NULL;
      LengthSwUpAdhesionFault = FALSE;
      LengthSwDownAdhesionFault = FALSE;
      du:
      LengthSwTimer = GetCurMsTs();
    (default) -> LengthSwitchErrorDeal.Invalid
    LengthSwitchErrorDeal.Invalid -> LengthSwitchErrorDeal.Valid : /*开关有效  */
        | [enSeatMoveCmd.EN_NULL != MtrCtrlFault_DRLengthSwitch]
    LengthSwitchErrorDeal.Valid -> LengthSwitchErrorDeal.Invalid [order 1] : /* 跳变 无效 */
        | [enSeatMoveCmd.EN_NULL == MtrCtrlFault_DRLengthSwitch ...
        | || hasChanged(MtrCtrlFault_DRLengthSwitch)]
  state BackSwitchErrorDeal [parallel]
    settings: executionOrder=3
    state Valid
      (default) -> (junction 457)
      BackSwitchErrorDeal.Valid -> (junction 457) [order 1]
      (junction 457) -> (junction 458) [order 1] : /*持续有效时间超过90s，则诊断为开关粘滞故障*/
          | [TimeDiffTs(BackSwTimer,GetCurMsTs()) >= CAL_ManualSwValid_90s]
      (junction 457) -> (junction 464) [order 2] : {BackSwCmd = MtrCtrlFault_DRBackSwitch;
          | BackSwUpAdhesionFault = FALSE;
          | BackSwDownAdhesionFault = FALSE;}
      (junction 458) -> (junction 465) : {BackSwCmd = enSeatMoveCmd.EN_NULL;
          | BackSwTimer = GetDefTime(CAL_ManualSwValid_90s,GetCurMsTs());
          | BackSwAdhesionFault = TRUE;}
      (junction 465) -> (junction 470) [order 1] : [enSeatMoveCmd.EN_UP_FORWARD == MtrCtrlFault_DRBackSwitch]
      (junction 465) -> (junction 461) [order 2] : {BackSwDownAdhesionFault = TRUE;}
      (junction 470) -> (junction 469) : {BackSwUpAdhesionFault = TRUE;}
      (junction 461) -> (junction 464)
      (junction 469) -> (junction 461)
      (junction 464) -> (junction 463)
    state Invalid
      en:
      BackSwTimer = GetCurMsTs();
      BackSwAdhesionFault = FALSE;
      BackSwCmd = enSeatMoveCmd.EN_NULL;
      BackSwUpAdhesionFault = FALSE;
      BackSwDownAdhesionFault = FALSE;
      du:
      BackSwTimer = GetCurMsTs();
    (default) -> BackSwitchErrorDeal.Invalid
    BackSwitchErrorDeal.Invalid -> BackSwitchErrorDeal.Valid : /*开关有效  */
        | [enSeatMoveCmd.EN_NULL != MtrCtrlFault_DRBackSwitch]
    BackSwitchErrorDeal.Valid -> BackSwitchErrorDeal.Invalid [order 1] : /* 跳变 无效 */
        | [enSeatMoveCmd.EN_NULL == MtrCtrlFault_DRBackSwitch ...
        | || hasChanged(MtrCtrlFault_DRBackSwitch)]
  state FrontSwitchErrorDeal [parallel]
    settings: executionOrder=4
    state Valid
      (default) -> (junction 485)
      FrontSwitchErrorDeal.Valid -> (junction 485) [order 1]
      (junction 485) -> (junction 486) [order 1] : /*持续有效时间超过90s，则诊断为开关粘滞故障*/
          | [TimeDiffTs(FrontSwTimer,GetCurMsTs()) >= CAL_ManualSwValid_90s]
      (junction 485) -> (junction 492) [order 2] : {FrontSwCmd = MtrCtrlFault_DRFrontSwitch;
          | FrontSwUpAdhesionFault = FALSE;
          | FrontSwDownAdhesionFault = FALSE;}
      (junction 486) -> (junction 493) : {FrontSwCmd = enSeatMoveCmd.EN_NULL;
          | FrontSwTimer = GetDefTime(CAL_ManualSwValid_90s,GetCurMsTs());
          | FrontSwAdhesionFault = TRUE;}
      (junction 493) -> (junction 498) [order 1] : [enSeatMoveCmd.EN_UP_FORWARD == MtrCtrlFault_DRFrontSwitch]
      (junction 493) -> (junction 489) [order 2] : {FrontSwDownAdhesionFault = TRUE;}
      (junction 498) -> (junction 497) : {FrontSwUpAdhesionFault = TRUE;}
      (junction 489) -> (junction 492)
      (junction 497) -> (junction 489)
      (junction 492) -> (junction 491)
    state Invalid
      en:
      FrontSwTimer = GetCurMsTs();
      FrontSwAdhesionFault = FALSE;
      FrontSwCmd = enSeatMoveCmd.EN_NULL;
      FrontSwUpAdhesionFault = FALSE;
      FrontSwDownAdhesionFault = FALSE;
      du:
      FrontSwTimer = GetCurMsTs();
    (default) -> FrontSwitchErrorDeal.Invalid
    FrontSwitchErrorDeal.Invalid -> FrontSwitchErrorDeal.Valid : /*开关有效  */
        | [enSeatMoveCmd.EN_NULL != MtrCtrlFault_DRFrontSwitch]
    FrontSwitchErrorDeal.Valid -> FrontSwitchErrorDeal.Invalid [order 1] : /* 跳变 无效 */
        | [enSeatMoveCmd.EN_NULL == MtrCtrlFault_DRFrontSwitch ...
        | || hasChanged(MtrCtrlFault_DRFrontSwitch)]
  data: Ts function_output; lastTs function_input; Ts function_input; OutTs function_output; DefTs function_input; Ts function_input; OutTs function_output; MtrCtrlFault_DRHeightSwitch input; MtrCtrlFault_DRLengthSwitch input; MtrCtrlFault_DRBackSwitch input; MtrCtrlFault_DRFrontSwitch input; HeightSwAdhesionFault output uint8; LengthSwAdhesionFault output uint8; BackSwAdhesionFault output uint8; FrontSwAdhesionFault output uint8; HeightSwTimer local uint32; TRUE parameter; FALSE parameter; LengthSwTimer local uint32; BackSwTimer local uint32; FrontSwTimer local uint32; CAL_ManualSwValid_90s parameter; HeightSwCmd output Enum: enSeatMoveCmd; LengthSwCmd output Enum: enSeatMoveCmd; BackSwCmd output Enum: enSeatMoveCmd; FrontSwCmd output Enum: enSeatMoveCmd; HeightSwUpAdhesionFault output uint8; HeightSwDownAdhesionFault output uint8; LengthSwUpAdhesionFault output uint8; LengthSwDownAdhesionFault output uint8; BackSwUpAdhesionFault output uint8; BackSwDownAdhesionFault output uint8; FrontSwUpAdhesionFault output uint8; FrontSwDownAdhesionFault output uint8
